simulink model "CRDI_LPP"  (R2019a)
settings: Solver=FixedStepDiscrete  StartTime=0.0  StopTime=10  FixedStep=0.01  RelTol=1e-3
libraries: simulink x2
settings Model: DataDictionary=CRDI_LPP.sldd  Creator=suraj  LastModifiedBy=suraj
settings DebuggingCC: InheritedTsInSrcMsg=none
settings ConfigComp: CovEnable=on  RecordCoverage=on  CovMetricSettings=dcmwe  CovModelRefEnable=on  DVTestSuiteOptimization=Auto  DVDetectDeadLogic=on  DVDetectActiveLogic=on  DVDetectOutOfBounds=on  DVRebuildModelRepresentation=Always

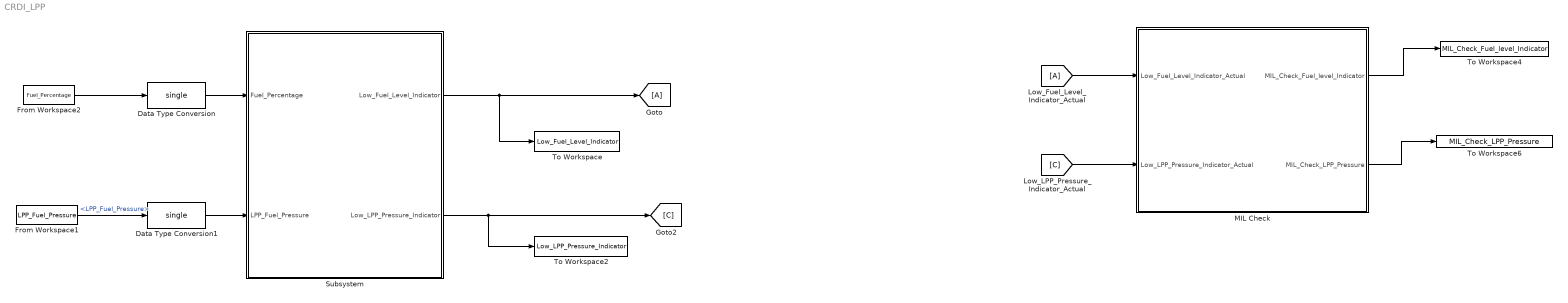
== system CRDI_LPP ==
  Data Type Conversion : DataTypeConversion  OutDataTypeStr=single
  Data Type Conversion1 : DataTypeConversion  OutDataTypeStr=single
  From Workspace1 : FromWorkspace  VariableName=LPP_Fuel_Pressure  OutDataTypeStr=double  SampleTime=0
  From Workspace2 : FromWorkspace  VariableName=Fuel_Percentage  SampleTime=0
  MIL Check : Subsystem
  Subsystem : Subsystem  TreatAsAtomicUnit=on
  To Workspace : ToWorkspace  VariableName=Low_Fuel_Level_Indicator  SaveFormat=Timeseries  SampleTime=-1
  To Workspace2 : ToWorkspace  VariableName=Low_LPP_Pressure_Indicator  SaveFormat=Timeseries  SampleTime=-1
  To Workspace4 : ToWorkspace  VariableName=MIL_Check_Fuel_level_Indicator  SaveFormat=Timeseries  SampleTime=-1
  To Workspace6 : ToWorkspace  VariableName=MIL_Check_LPP_Pressure  SaveFormat=Timeseries  SampleTime=-1
  wires:
  Subsystem/1(Low_Fuel_Level_Indicator) -> [A], To Workspace/1
  From Workspace1/1 -> Data Type Conversion1/1  "<LPP_Fuel_Pressure>"
  Subsystem/2(Low_LPP_Pressure_Indicator) -> To Workspace2/1, [C]
  [A] -> MIL Check/1(Low_Fuel_Level_Indicator_Actual)
  [C] -> MIL Check/2(Low_LPP_Pressure_Indicator_Actual)
  MIL Check/2(MIL_Check_LPP_Pressure) -> To Workspace6/1
  MIL Check/1(MIL_Check_Fuel_level_Indicator) -> To Workspace4/1
  Data Type Conversion/1 -> Subsystem/1(Fuel_Percentage)
  Data Type Conversion1/1 -> Subsystem/2(LPP_Fuel_Pressure)
  From Workspace2/1 -> Data Type Conversion/1

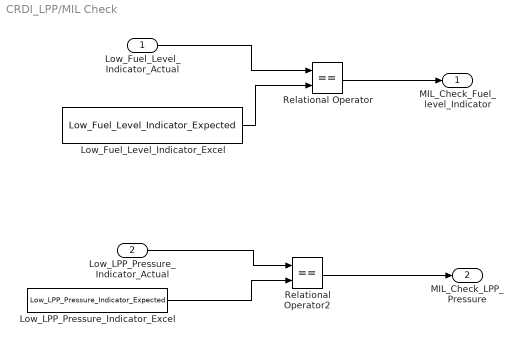
== system CRDI_LPP/MIL Check ==
  Low_Fuel_Level_Indicator_Actual : Inport
  Low_LPP_Pressure_Indicator_Actual : Inport  Port=2
  "Low_Fuel_Level_Indicator_Excel " : FromWorkspace  VariableName=Low_Fuel_Level_Indicator_Expected  SampleTime=0
  Low_LPP_Pressure_Indicator_Excel : FromWorkspace  VariableName=Low_LPP_Pressure_Indicator_Expected  SampleTime=0
  Relational Operator : RelationalOperator  Operator===  OutDataTypeStr=boolean  RndMeth=Simplest
  Relational Operator2 : RelationalOperator  Operator===  OutDataTypeStr=boolean  RndMeth=Simplest
  MIL_Check_Fuel_level_Indicator : Outport
  MIL_Check_LPP_Pressure : Outport  Port=2
  wires:
  Low_Fuel_Level_Indicator_Actual/1 -> Relational Operator/1
  "Low_Fuel_Level_Indicator_Excel "/1 -> Relational Operator/2
  Relational Operator/1 -> MIL_Check_Fuel_level_Indicator/1
  Low_LPP_Pressure_Indicator_Actual/1 -> Relational Operator2/1
  Low_LPP_Pressure_Indicator_Excel/1 -> Relational Operator2/2
  Relational Operator2/1 -> MIL_Check_LPP_Pressure/1

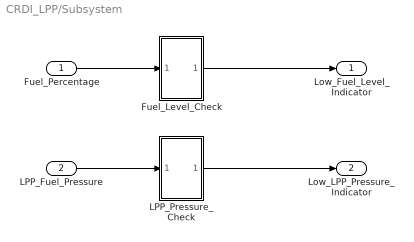
== system CRDI_LPP/Subsystem ==
  Fuel_Percentage : Inport  OutDataTypeStr=single
  LPP_Fuel_Pressure : Inport  Port=2  OutDataTypeStr=single
  Fuel_Level_Check : Subsystem
  LPP_Pressure_Check : Subsystem
  Low_Fuel_Level_Indicator : Outport
  Low_LPP_Pressure_Indicator : Outport  Port=2
  wires:
  LPP_Fuel_Pressure/1 -> LPP_Pressure_Check/1(In1)
  Fuel_Percentage/1 -> Fuel_Level_Check/1(In1)
  Fuel_Level_Check/1(Out1) -> Low_Fuel_Level_Indicator/1
  LPP_Pressure_Check/1(Out1) -> Low_LPP_Pressure_Indicator/1

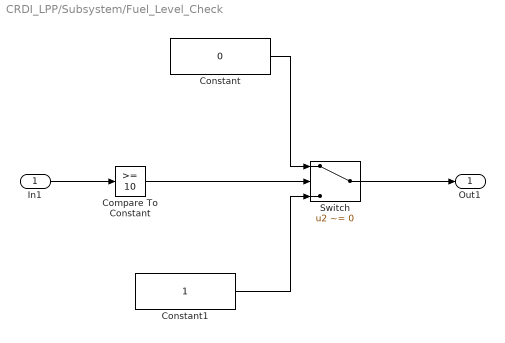
== system CRDI_LPP/Subsystem/Fuel_Level_Check ==
  In1 : Inport  OutDataTypeStr=single
  Compare To Constant : simulink/Logic and Bit Operations/Compare To Constant  relop=>=  const=10  OutDataTypeStr=boolean
  Constant : Constant  Value=0  OutDataTypeStr=boolean
  Constant1 : Constant  OutDataTypeStr=boolean
  Switch : Switch  Criteria=u2 ~= 0  OutDataTypeStr=boolean
  Out1 : Outport  OutDataTypeStr=boolean
  wires:
  Switch/1 -> Out1/1
  Constant1/1 -> Switch/3
  Constant/1 -> Switch/1
  Compare To Constant/1 -> Switch/2
  In1/1 -> Compare To Constant/1

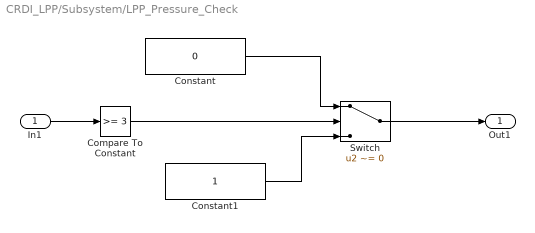
== system CRDI_LPP/Subsystem/LPP_Pressure_Check ==
  In1 : Inport  OutDataTypeStr=single
  Compare To Constant : simulink/Logic and Bit Operations/Compare To Constant  relop=>=  const=3  OutDataTypeStr=boolean
  Constant : Constant  Value=0  OutDataTypeStr=single
  Constant1 : Constant  OutDataTypeStr=single
  Switch : Switch  Criteria=u2 ~= 0  OutDataTypeStr=boolean
  Out1 : Outport  OutDataTypeStr=boolean
  wires:
  In1/1 -> Compare To Constant/1
  Compare To Constant/1 -> Switch/2
  Constant/1 -> Switch/1
  Constant1/1 -> Switch/3
  Switch/1 -> Out1/1
